simulink model "CDPR_simulation_w_motor"  (R2023b)
settings: Solver=ode15s  StartTime=0.0  StopTime=10.0  RelTol=1e-3
values from neighbouring files (symbols this model uses):
  A = 1e-6    (= 1e-06)    [init.m]
  a = [a1 a2 a3 a4]    [init.m]
  A_c_aug = [A_c    zeros(6,6) ... (first row only)    [init.m]
  b = [b1 b2 b3 b4]    [init.m]
  B_c_aug = [B_c; zeros(6,3)]    [init.m]
  d_c = [ 0 ... (first row only)    [init.m]
  d_c_aug = [d_c; zeros(6,1)]    [init.m]
  E = 100E9    (= 100000000000)    [init.m]
  f_max = 100    [init.m]
  f_min = 10    [init.m]
  f_ref = 25    [init.m]
  I_gain_f = 10    [init.m]
  Izz = 6.25e-4    (= 0.000625)    [init.m]
  K_a = [diag([-10,-10,-1]) zeros(3,3)]    [init.m]
  K_d = B_c\eye(6)    [init.m]
  K_f = [180*diag([1,1,1]) 10*diag([1,1,1])]    [init.m]
  K_r = pinv((B_c*K_f-A_c)\B_c)    [init.m]
  ln0 = zeros(size(b,2),1)    [init.m]
  mp = 0.250    (= 0.25)    [init.m]
  P_gain_f = 75    [init.m]
  q0 = [r0; theta0]    [init.m]
  qd0 = [xd0;yd0; thetad0]    [init.m]
  w = [ 0 ... (first row only)    [init.m]
  zeroI = [zeros(6,6);eye(6)]    [init.m]
undefined symbols (not defined in the file or in its folder): Clarke, current_m_max, current_m_min, fourier_coeff_a, fourier_coeff_b, i_m_max, i_m_min, J_m, K_e, l_m, n_p_pairs, r_m, r_w, thetar0
libraries: slpidlib x1
settings Model: Creator=Sølve  LastModifiedBy=solvno
settings DebuggingCC: UnconnectedInputMsg=warning  UnconnectedOutputMsg=warning  UnconnectedLineMsg=warning
settings ModelReferenceCC: EnableRefExpFcnMdlSchedulingChecks=on
settings RTWCC: DLArmComputeVersion=19.05

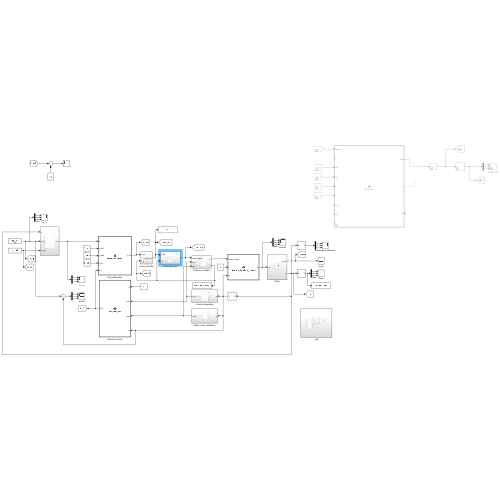
[thumbnail: Simulink's stored preview of the top-level diagram]
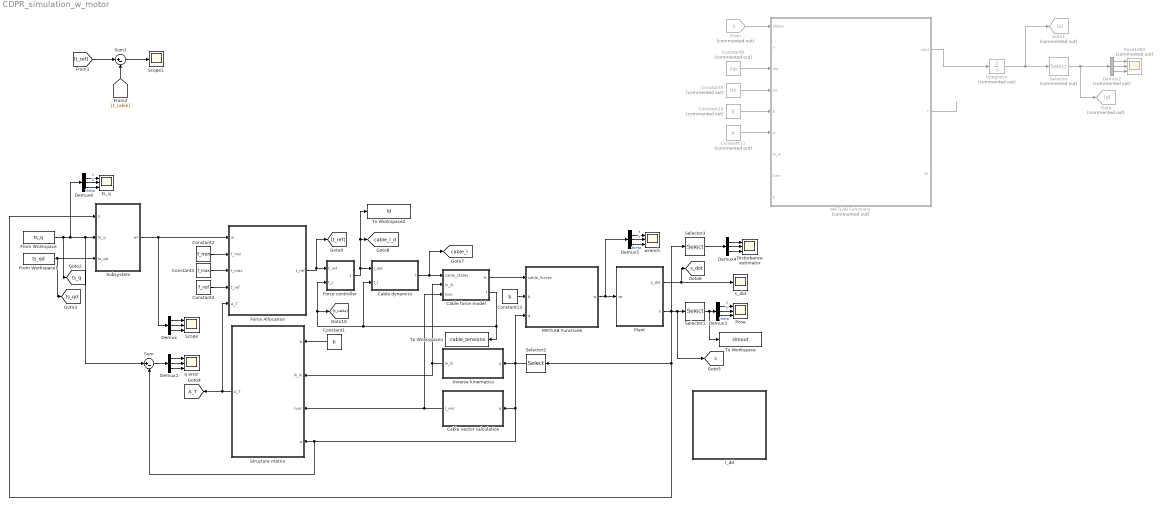
== system CDPR_simulation_w_motor ==
  Cable dynamics : Subsystem
  Cable force model : Subsystem
  Cable vector calculation : Subsystem
  Constant1 : Constant  Value=b
  Constant10 : Constant  Commented=on  Value=E
  Constant11 : Constant  Commented=on  Value=A
  Constant13 : Constant  Value=b
  Constant2 : Constant  Value=f_min
  Constant3 : Constant  Value=f_max
  Constant4 : Constant  Value=f_ref
  Constant8 : Constant  Commented=on  Value=mp
  Constant9 : Constant  Commented=on  Value=Izz
  Demux{,1,3..6} (6 alike) : Demux  Outputs=3
  Demux2 : Demux  Commented=on  Outputs=3
  Disturbance estimator : Scope  NumInputPorts=3
  Force Allocation : MATLAB Function  TreatAsAtomicUnit=on
  Force controller : Subsystem
  From : From  Commented=on  GotoTag=s
  From Workspace : FromWorkspace  VariableName=ts_q
  From Workspace1 : FromWorkspace  VariableName=ts_qd
  Goto : Goto  Commented=on  GotoTag=q
  Goto1 : Goto  Commented=on  GotoTag=s
  Integrator : Integrator  Commented=on  InitialCondition=[q0;qd0;ln0]
  Inverse kinematics : Subsystem
  MATLAB Function3 : MATLAB Function  Commented=on  TreatAsAtomicUnit=on
  MATLAB Function6 : MATLAB Function  TreatAsAtomicUnit=on
  Plant : Subsystem
  Pose : Scope  NumInputPorts=3
  Pose1000 : Scope  Commented=on  NumInputPorts=3
  Scope : Scope  NumInputPorts=3
  Scope1 : Scope
  Selector : Selector  Commented=on  InputPortWidth=10  IndexOptions=Index vector (dialog)  Indices=[1 2 3]  OutputSizes=1
  Selector1 : Selector  InputPortWidth=12  IndexOptions=Index vector (dialog)  Indices=[1 2 3]  OutputSizes=1
  Selector2 : Selector  InputPortWidth=12  IndexOptions=Index vector (dialog)  Indices=[1 2 3]  OutputSizes=1
  Selector3 : Selector  InputPortWidth=12  IndexOptions=Index vector (dialog)  Indices=[7 8 9]  OutputSizes=1
  Structure matrix : MATLAB Function  TreatAsAtomicUnit=on
  Subsystem : Subsystem
  Sum : Sum  Inputs=|+-
  Sum1 : Sum  Inputs=|+-
  To Workspace : ToWorkspace  VariableName=simout  SaveFormat=Timeseries  SampleTime=-1
  To Workspace1 : ToWorkspace  VariableName=cable_tensions  SaveFormat=Timeseries  SampleTime=-1
  To Workspace2 : ToWorkspace  VariableName=ld  SaveFormat=Timeseries  SampleTime=-1
  l_dd : Subsystem
  q error : Scope  NumInputPorts=3
  s_dot : Scope
  ts_q : Scope  NumInputPorts=3
  wrench : Scope  NumInputPorts=3
  tag scope: A_T=global, cable_l=global, cable_l_d=global, s=global, s_dot=global, ts_q=global, ts_qd=global
  wires:
  Constant1/1 -> Structure matrix/1(b)
  Constant2/1 -> Force Allocation/2(f_min)
  Constant4/1 -> Force Allocation/4(f_ref)
  Constant3/1 -> Force Allocation/3(f_max)
  Force Allocation/1(t_ref) -> Force controller/1(t_ref), [t_ref]
  Constant8/1 -> MATLAB Function3/3(mp)
  Constant9/1 -> MATLAB Function3/4(Izz)
  Constant10/1 -> MATLAB Function3/5(E)
  Constant11/1 -> MATLAB Function3/6(A)
  MATLAB Function3/2(t) -> ?
  MATLAB Function3/1(xdot) -> Integrator/1
  Integrator/1 -> Goto1/1, Selector/1
  Selector/1 -> Demux2/1, Goto/1
  From/1 -> MATLAB Function3/1(states)
  Inverse kinematics/1(ln_ik) -> Structure matrix/2(ln_ik), Cable force model/2(ln_ik)
  Demux/1 -> Scope/1
  Demux/2 -> Scope/2
  Demux/3 -> Scope/3
  Demux1/1 -> q error/1
  Demux1/3 -> q error/3
  Demux1/2 -> q error/2
  Selector2/1 -> Sum/2, Structure matrix/4(q), Cable vector calculation/1(q), MATLAB Function6/3(q), Inverse kinematics/1(q)
  Sum/1 -> Demux1/1
  Demux2/1 -> Pose1000/1
  Demux2/2 -> Pose1000/2
  Demux2/3 -> Pose1000/3
  Plant/2(s) -> Selector3/1, [s], Selector1/1, Subsystem/1(s), Selector2/1
  Demux3/3 -> Pose/3  "theta"
  Demux3/2 -> Pose/2  "y"
  Demux3/1 -> Pose/1  "x"
  Plant/1(s_dot) -> [s_dot], s_dot/1
  Constant13/1 -> MATLAB Function6/2(b)
  Cable force model/1(fc) -> MATLAB Function6/1(cable_forces)
  Cable dynamics/1(l) -> [cable_l], Cable force model/1(cable_states)
  Cable force model/2(t) -> Cable dynamics/2(t_l), Force controller/2(t_c), [t_cable], To Workspace1/1
  Cable vector calculation/1(l_vec) -> Cable force model/3(lvec), Structure matrix/3(lvec)
  Structure matrix/1(A_T) -> [A_T], Force Allocation/5(A_T)
  Selector1/1 -> To Workspace/1, Demux3/1
  Subsystem/1(wr) -> Demux/1, Force Allocation/1(w)
  From Workspace1/1 -> [ts_qd], Subsystem/3(ts_qd)
  Selector3/1 -> Demux4/1
  Demux4/1 -> Disturbance estimator/1
  Demux4/2 -> Disturbance estimator/2
  Demux4/3 -> Disturbance estimator/3
  Demux5/1 -> wrench/1  "x"
  Demux5/3 -> wrench/3  "theta"
  Demux5/2 -> wrench/2  "y"
  MATLAB Function6/1(w) -> Demux5/1, Plant/1(wr)
  [t_cable] -> Sum1/2
  [t_ref] -> Sum1/1
  Sum1/1 -> Scope1/1
  Force controller/1(l_dot_ref) -> To Workspace2/1, [cable_l_d], Cable dynamics/1(l_dot)
  Demux6/1 -> ts_q/1  "x"
  Demux6/3 -> ts_q/3  "theta"
  Demux6/2 -> ts_q/2  "y"
  From Workspace/1 -> Demux6/1, Subsystem/2(ts_q), Sum/1, [ts_q]

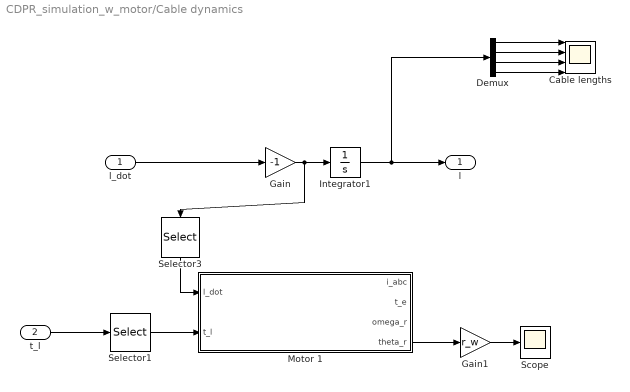
== system CDPR_simulation_w_motor/Cable dynamics ==
  l_dot : Inport
  t_l : Inport  Port=2
  Cable lengths : Scope  NumInputPorts=4
  Demux : Demux
  Gain : Gain  Gain=-1
  Gain1 : Gain  Gain=r_w
  Integrator1 : Integrator  InitialCondition=ln0
  Motor 1 : Subsystem
  Scope : Scope
  Selector1 : Selector  InputPortWidth=4  IndexOptions=Index vector (dialog)  Indices=[1]  OutputSizes=1
  Selector3 : Selector  InputPortWidth=4  IndexOptions=Index vector (dialog)  Indices=[1]  OutputSizes=1
  l : Outport
  wires:
  Integrator1/1 -> Demux/1, l/1
  l_dot/1 -> Gain/1
  Gain/1 -> Selector3/1, Integrator1/1
  Demux/1 -> Cable lengths/1
  Demux/2 -> Cable lengths/2
  Demux/3 -> Cable lengths/3
  Demux/4 -> Cable lengths/4
  t_l/1 -> Selector1/1
  Motor 1/4(theta_r) -> Gain1/1
  Gain1/1 -> Scope/1
  Selector3/1 -> Motor 1/1(l_dot)
  Selector1/1 -> Motor 1/2(t_l)

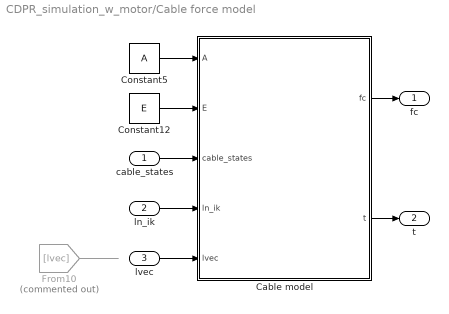
== system CDPR_simulation_w_motor/Cable force model ==
  cable_states : Inport
  ln_ik : Inport  Port=2
  lvec : Inport  Port=3
  Cable model : MATLAB Function  TreatAsAtomicUnit=on
  Constant12 : Constant  Value=E
  Constant5 : Constant  Value=A
  From10 : From  Commented=on  GotoTag=lvec  TagVisibility=global
  fc : Outport
  t : Outport  Port=2
  wires:
  Constant12/1 -> Cable model/2(E)
  From10/1 -> ?
  ln_ik/1 -> Cable model/4(ln_ik)
  Constant5/1 -> Cable model/1(A)
  Cable model/2(t) -> t/1
  cable_states/1 -> Cable model/3(cable_states)
  Cable model/1(fc) -> fc/1
  lvec/1 -> Cable model/5(lvec)

== system CDPR_simulation_w_motor/Cable vector calculation ==
  q : Inport
  Constant : Constant  Value=b
  Constant5 : Constant  Value=a
  MATLAB Function5 : MATLAB Function  TreatAsAtomicUnit=on
  l_vec : Outport
  wires:
  Constant/1 -> MATLAB Function5/3(b)
  q/1 -> MATLAB Function5/1(q)
  Constant5/1 -> MATLAB Function5/2(a)
  MATLAB Function5/1(l_vec) -> l_vec/1

== system CDPR_simulation_w_motor/Force controller ==
  t_ref : Inport
  t_c : Inport  Port=2
  PID Controller (2DOF) : slpidlib/PID Controller (2DOF)  Controller=PI  Form=Parallel  TimeDomain=Continuous-time  UseExternalTs=off  SampleTime=-1  IntegratorMethod=Forward Euler  FilterMethod=Forward Euler  ControllerParametersSource=internal  P=P_gain_f  I=I_gain_f  UseKiTs=off  D=5  N=100  UseFilter=on  b=1  c=1  TunerSelectOption=Transfer Function Based (PID Tuner App)  InitialConditionSource=internal  InitialConditionForIntegrator=0  InitialConditionForFilter=0  DifferentiatorICPrevScaledInput=0  ExternalReset=none  TrackingMode=off  Kt=1  LimitOutput=off  SatLimitsSource=internal  UpperSaturationLimit=inf  LowerSaturationLimit=-inf  LinearizeAsGain=on  AntiWindupMode=none  Kb=1  LimitIntegrator=off  UpperIntegratorSaturationLimit=inf  LowerIntegratorSaturationLimit=-inf  POutMin=[]  POutMax=[]  IOutMin=[]  IOutMax=[]  DOutMin=[]  DOutMax=[]  NOutMin=[]  NOutMax=[]  bOutMin=[]  bOutMax=[]  cOutMin=[]  cOutMax=[]  SumOutMin=[]  SumOutMax=[]  SaturationOutMin=[]  SaturationOutMax=[]  PParamMin=[]  PParamMax=[]  IParamMin=[]  IParamMax=[]  DParamMin=[]  DParamMax=[]  NParamMin=[]  NParamMax=[]  bParamMin=[]  bParamMax=[]  cParamMin=[]  cParamMax=[]  KbParamMin=[]  KbParamMax=[]  KtParamMin=[]  KtParamMax=[]  KbOutMin=[]  KbOutMax=[]  KtOutMin=[]  KtOutMax=[]  IntegratorOutMin=[]  IntegratorOutMax=[]  FilterOutMin=[]  FilterOutMax=[]  SumI1OutMin=[]  SumI1OutMax=[]  SumI2OutMin=[]  SumI2OutMax=[]  SumI3OutMin=[]  SumI3OutMax=[]  SumI4OutMin=[]  SumI4OutMax=[]  SumDOutMin=[]  SumDOutMax=[]  Sum1OutMin=[]  Sum1OutMax=[]  Sum2OutMin=[]  Sum2OutMax=[]  Sum3OutMin=[]  Sum3OutMax=[]  DifferentiatorOutMin=[]  DifferentiatorOutMax=[]  FilterDiffOutCoefMin=[]  FilterDiffOutCoefMax=[]  ReciprocalOutMin=[]  ReciprocalOutMax=[]  SumDenOutMin=[]  SumDenOutMax=[]  SumNumOutMin=[]  SumNumOutMax=[]  DivideOutMin=[]  DivideOutMax=[]  UdiffTsProdOutMin=[]  UdiffTsProdOutMax=[]  NTsProdOutMin=[]  NTsProdOutMax=[]  UintegralTsProdOutMin=[]  UintegralTsProdOutMax=[]  UngainTsProdOutMin=[]  UngainTsProdOutMax=[]  ClampingZeroOutDataTypeStr=Inherit: Inherit via back propagation  ClampingZeroOutMin=[]  ClampingZeroOutMax=[]  FilterDenConstantOutDataTypeStr=Inherit: Inherit via back propagation  FilterDenConstantOutMin=[]  FilterDenConstantOutMax=[]  PCopyOutDataTypeStr=Inherit: Inherit via back propagation  PCopyOutMin=[]  PCopyOutMax=[]  NCopyOutDataTypeStr=Inherit: Inherit via back propagation  NCopyOutMin=[]  NCopyOutMax=[]  IntegratorContinuousStateAttributes=''  IntegratorStateMustResolveToSignalObject=off  IntegratorRTWStateStorageClass=Auto  FilterContinuousStateAttributes=''  FilterStateMustResolveToSignalObject=off  FilterRTWStateStorageClass=Auto  ParallelPVariant=InternalParameters  IdealPVariant=Disabled  IVariant=InternalParameters  DVariant=Disabled  bVariant=InternalParameters  cVariant=Disabled  IntegratorVariant=Continuous  SatVariant=Disabled  AWVariant=Passthrough  PCopyVariant=Disabled  TRVariant=Disabled  FdbkBlocksVariant=Forward  IdealPFdbkVariant=Disabled  SatFdbkVariant=Disabled  DerivativeFilterVariant=Disabled  NVariant=Disabled  NCopyVariant=Disabled_SignalSpec  FilterICVariant=Disabled  IntegratorICVariant=InternalICs  ExternalResetVariant=Disabled  TRSumVariant=Passthrough  SumFdbkVariant=Disabled  SumVariant=Sum_PI  TsampFilterVariant=InternalTs  TsampNgainVariant=Passthrough  TsampIntegralVariant=Disabled_SignalSpec  ExternalSaturationOutDataTypeStr=Inherit: Same as second input
  Saturation : Saturate  UpperLimit=5  LowerLimit=-5
  l_dot_ref : Outport
  wires:
  t_ref/1 -> PID Controller (2DOF)/1
  t_c/1 -> PID Controller (2DOF)/2
  PID Controller (2DOF)/1 -> Saturation/1
  Saturation/1 -> l_dot_ref/1

== system CDPR_simulation_w_motor/Inverse kinematics ==
  q : Inport
  Constant6 : Constant  Value=a
  Constant7 : Constant  Value=b
  MATLAB Function4 : MATLAB Function  TreatAsAtomicUnit=on
  ln_ik : Outport
  wires:
  MATLAB Function4/1(ln) -> ln_ik/1
  Constant6/1 -> MATLAB Function4/2(a)
  q/1 -> MATLAB Function4/1(q)
  Constant7/1 -> MATLAB Function4/3(b)

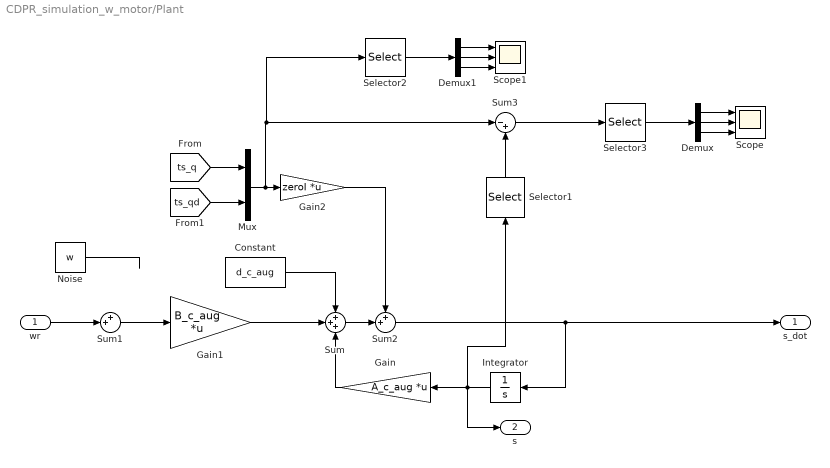
== system CDPR_simulation_w_motor/Plant ==
  wr : Inport
  Constant : Constant  Value=d_c_aug
  Demux : Demux  Outputs=3
  Demux1 : Demux  Outputs=3
  Gain : Gain  Gain=A_c_aug  Multiplication=Matrix(K*u)
  Gain1 : Gain  Gain=B_c_aug  Multiplication=Matrix(K*u)
  Gain2 : Gain  Gain=zeroI  Multiplication=Matrix(K*u)
  Integrator : Integrator  InitialCondition=[q0;qd0; zeros(6,1)]
  Mux : Mux  Inputs=2
  Noise : Constant  Value=w
  Scope : Scope  NumInputPorts=3
  Scope1 : Scope  NumInputPorts=3
  Selector1 : Selector  InputPortWidth=12  IndexOptions=Index vector (dialog)  Indices=[1 2 3 4 5 6]  OutputSizes=1
  Selector2 : Selector  InputPortWidth=6  IndexOptions=Index vector (dialog)  Indices=[1 2 3]  OutputSizes=1
  Selector3 : Selector  InputPortWidth=6  IndexOptions=Index vector (dialog)  Indices=[1 2 3]  OutputSizes=1
  Sum : Sum  Inputs=+++
  Sum1 : Sum  Inputs=++|
  Sum2 : Sum  Inputs=++|
  Sum3 : Sum  Inputs=|-+
  s_dot : Outport
  s : Outport  Port=2
  wires:
  Integrator/1 -> Selector1/1, s/1, Gain/1
  wr/1 -> Sum1/2
  Constant/1 -> Sum/1
  Gain1/1 -> Sum/2
  Gain/1 -> Sum/3
  Sum2/1 -> Integrator/1, s_dot/1
  [ts_q] -> Mux/1
  [ts_qd] -> Mux/2
  Sum1/1 -> Gain1/1
  Noise/1 -> ?
  Sum/1 -> Sum2/2
  Gain2/1 -> Sum2/1
  Sum3/1 -> Selector3/1
  Demux/1 -> Scope/1
  Demux/2 -> Scope/2
  Demux/3 -> Scope/3
  Selector3/1 -> Demux/1
  Selector1/1 -> Sum3/2
  Demux1/3 -> Scope1/3
  Selector2/1 -> Demux1/1
  Demux1/2 -> Scope1/2
  Demux1/1 -> Scope1/1
  Mux/1 -> Selector2/1, Sum3/1, Gain2/1

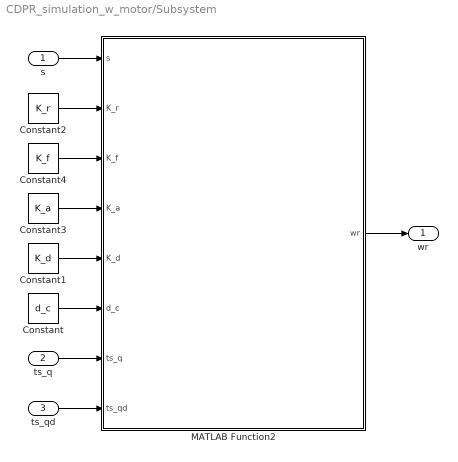
== system CDPR_simulation_w_motor/Subsystem ==
  s : Inport
  ts_q : Inport  Port=2
  ts_qd : Inport  Port=3
  Constant : Constant  Value=d_c
  Constant1 : Constant  Value=K_d
  Constant2 : Constant  Value=K_r
  Constant3 : Constant  Value=K_a
  Constant4 : Constant  Value=K_f
  MATLAB Function2 : MATLAB Function  TreatAsAtomicUnit=on
  wr : Outport
  wires:
  ts_q/1 -> MATLAB Function2/7(ts_q)
  ts_qd/1 -> MATLAB Function2/8(ts_qd)
  MATLAB Function2/1(wr) -> wr/1
  s/1 -> MATLAB Function2/1(s)
  Constant/1 -> MATLAB Function2/6(d_c)
  Constant1/1 -> MATLAB Function2/5(K_d)
  Constant2/1 -> MATLAB Function2/2(K_r)
  Constant3/1 -> MATLAB Function2/4(K_a)
  Constant4/1 -> MATLAB Function2/3(K_f)

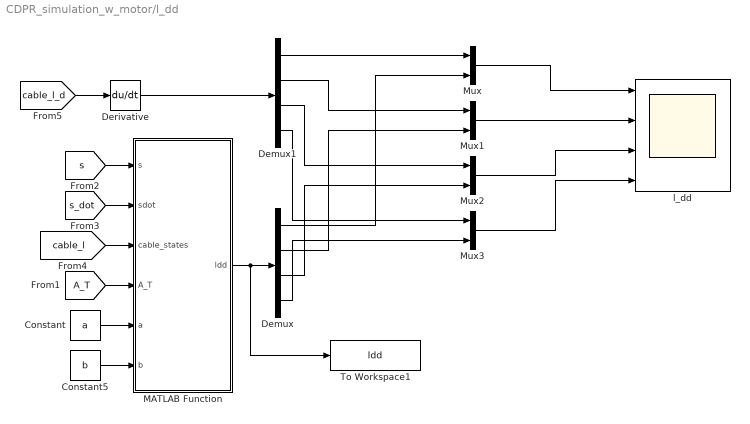
== system CDPR_simulation_w_motor/l_dd ==
  Constant : Constant  Value=a
  Constant5 : Constant  Value=b
  Demux : Demux
  Demux1 : Demux
  Derivative : Derivative  CoefficientInTFapproximation=0.0001
  MATLAB Function : MATLAB Function  TreatAsAtomicUnit=on
  Mux{,1..3} (4 alike) : Mux  Inputs=2
  To Workspace1 : ToWorkspace  VariableName=ldd  SaveFormat=Timeseries  SampleTime=-1
  l_dd : Scope  NumInputPorts=4
  wires:
  Constant/1 -> MATLAB Function/5(a)
  [A_T] -> MATLAB Function/4(A_T)
  [cable_l_d] -> Derivative/1
  Constant5/1 -> MATLAB Function/6(b)
  [s] -> MATLAB Function/1(s)
  [cable_l] -> MATLAB Function/3(cable_states)
  [s_dot] -> MATLAB Function/2(sdot)
  MATLAB Function/1(ldd) -> To Workspace1/1, Demux/1
  Derivative/1 -> Demux1/1
  Demux1/1 -> Mux/1
  Demux/1 -> Mux/2
  Demux1/2 -> Mux1/1
  Demux/2 -> Mux1/2
  Demux/3 -> Mux2/2
  Demux1/3 -> Mux2/1
  Demux1/4 -> Mux3/1
  Demux/4 -> Mux3/2
  Mux/1 -> l_dd/1
  Mux1/1 -> l_dd/2
  Mux2/1 -> l_dd/3
  Mux3/1 -> l_dd/4

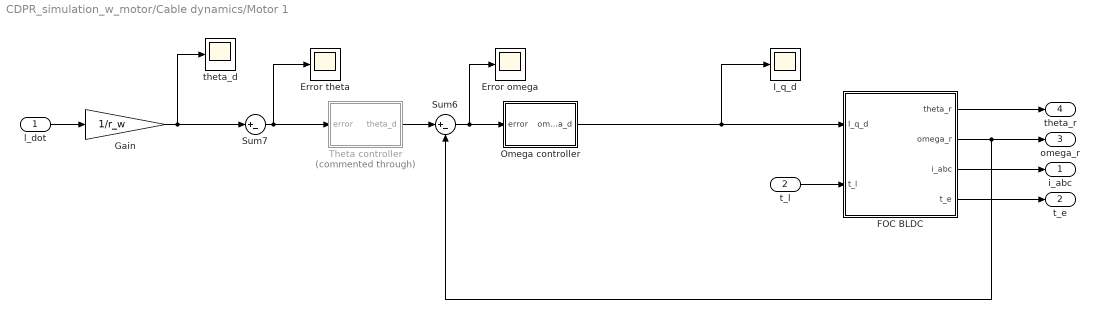
== system CDPR_simulation_w_motor/Cable dynamics/Motor 1 ==
  l_dot : Inport
  t_l : Inport  Port=2
  Error omega : Scope
  Error theta : Scope
  FOC BLDC : Subsystem
  Gain : Gain  Gain=1/r_w
  I_q_d : Scope
  Omega controller : Subsystem
  Sum6 : Sum  Inputs=|+-
  Sum7 : Sum  Inputs=|+-
  Theta controller : Subsystem  Commented=through
  theta_d : Scope
  i_abc : Outport
  t_e : Outport  Port=2
  omega_r : Outport  Port=3
  theta_r : Outport  Port=4
  wires:
  FOC BLDC/2(omega_r) -> Sum6/2, omega_r/1
  FOC BLDC/3(i_abc) -> i_abc/1
  Sum7/1 -> Theta controller/1(error), Error theta/1
  Sum6/1 -> Omega controller/1(error), Error omega/1
  FOC BLDC/1(theta_r) -> theta_r/1
  Theta controller/1(theta_d) -> Sum6/1
  FOC BLDC/4(t_e) -> t_e/1
  Omega controller/1(omega_d) -> I_q_d/1, FOC BLDC/1(I_q_d)
  l_dot/1 -> Gain/1
  t_l/1 -> FOC BLDC/2(t_l)
  Gain/1 -> theta_d/1, Sum7/1

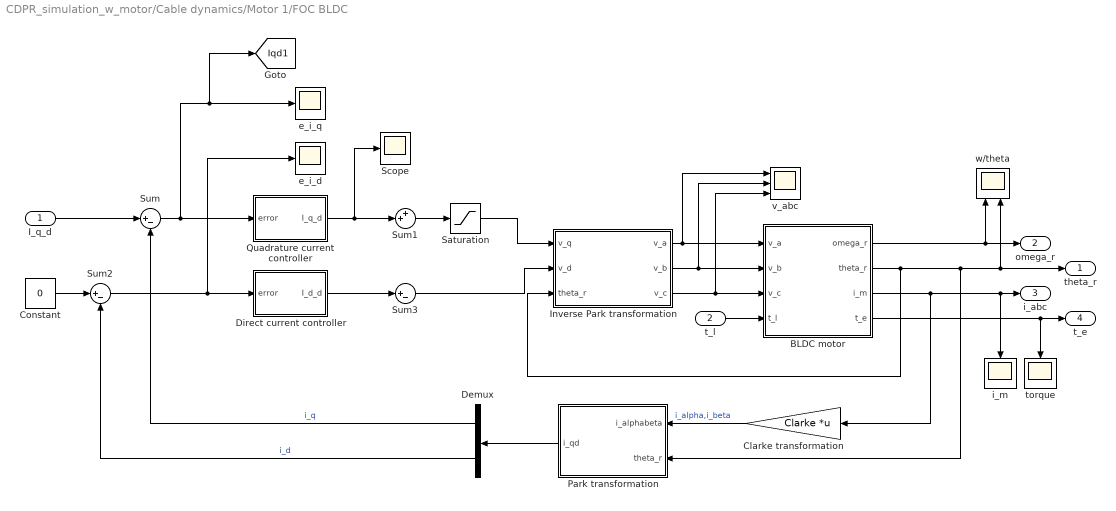
== system CDPR_simulation_w_motor/Cable dynamics/Motor 1/FOC BLDC ==
  I_q_d : Inport
  t_l : Inport  Port=2
  BLDC motor : Subsystem
  Clarke transformation : Gain  Gain=Clarke  Multiplication=Matrix(K*u) (u vector)
  Constant : Constant  Value=0
  Demux : Demux  Outputs=2
  Direct current controller : Subsystem
  Inverse Park transformation : MATLAB Function  TreatAsAtomicUnit=on
  Park transformation : MATLAB Function  TreatAsAtomicUnit=on
  Quadrature current controller : Subsystem
  Saturation : Saturate  UpperLimit=i_m_max  LowerLimit=i_m_min
  Scope : Scope
  Sum : Sum  Inputs=|+-
  Sum1 : Sum  Inputs=++|
  Sum2 : Sum  Inputs=|+-
  Sum3 : Sum  Inputs=|+-
  e_i_d : Scope
  e_i_q : Scope
  i_m : Scope
  torque : Scope
  v_abc : Scope  NumInputPorts=3
  w/theta : Scope  NumInputPorts=2
  theta_r : Outport
  omega_r : Outport  Port=2
  i_abc : Outport  Port=3
  t_e : Outport  Port=4
  tag scope: Iqd1=global
  wires:
  Sum/1 -> Quadrature current controller/1(error), [Iqd1], e_i_q/1
  Quadrature current controller/1(I_q_d) -> Scope/1, Sum1/2
  Constant/1 -> Sum2/1
  Sum2/1 -> Direct current controller/1(error), e_i_d/1
  Direct current controller/1(I_d_d) -> Sum3/1
  Sum1/1 -> Saturation/1
  Sum3/1 -> Inverse Park transformation/2(v_d)
  Inverse Park transformation/1(v_a) -> v_abc/1, BLDC motor/1(v_a)
  Inverse Park transformation/2(v_b) -> v_abc/2, BLDC motor/2(v_b)
  Inverse Park transformation/3(v_c) -> v_abc/3, BLDC motor/3(v_c)
  t_l/1 -> BLDC motor/4(t_l)
  BLDC motor/1(omega_r) -> omega_r/1, w/theta/1
  Clarke transformation/1 -> Park transformation/1(i_alphabeta)  "i_alpha,i_beta"
  BLDC motor/2(theta_r) -> Park transformation/2(theta_r), theta_r/1, w/theta/2, Inverse Park transformation/3(theta_r)
  Park transformation/1(i_qd) -> Demux/1
  Demux/1 -> Sum/2  "i_q"
  Demux/2 -> Sum2/2  "i_d"
  BLDC motor/3(i_m) -> i_m/1, i_abc/1, Clarke transformation/1
  BLDC motor/4(t_e) -> torque/1, t_e/1
  I_q_d/1 -> Sum/1
  Saturation/1 -> Inverse Park transformation/1(v_q)

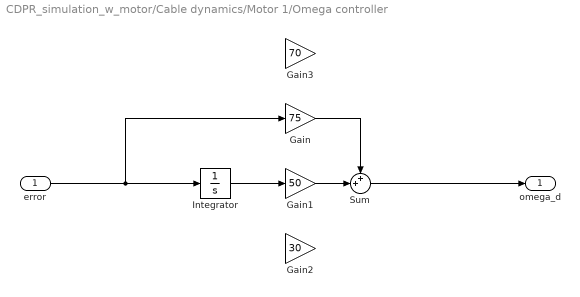
== system CDPR_simulation_w_motor/Cable dynamics/Motor 1/Omega controller ==
  error : Inport
  Gain : Gain  Gain=75
  Gain1 : Gain  Gain=50
  Gain2 : Gain  Gain=30
  Gain3 : Gain  Gain=70
  Integrator : Integrator
  Sum : Sum  Inputs=++|
  omega_d : Outport
  wires:
  Sum/1 -> omega_d/1
  Gain/1 -> Sum/1
  Gain1/1 -> Sum/2
  Integrator/1 -> Gain1/1
  error/1 -> Integrator/1, Gain/1

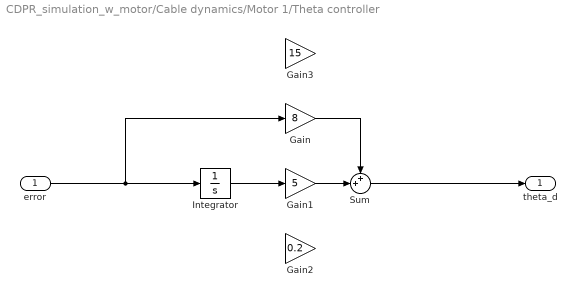
== system CDPR_simulation_w_motor/Cable dynamics/Motor 1/Theta controller ==
  error : Inport
  Gain : Gain  Gain=8
  Gain1 : Gain  Gain=5
  Gain2 : Gain  Gain=0.2
  Gain3 : Gain  Gain=15
  Integrator : Integrator
  Sum : Sum  Inputs=++|
  theta_d : Outport
  wires:
  error/1 -> Gain/1, Integrator/1
  Integrator/1 -> Gain1/1
  Gain1/1 -> Sum/2
  Gain/1 -> Sum/1
  Sum/1 -> theta_d/1

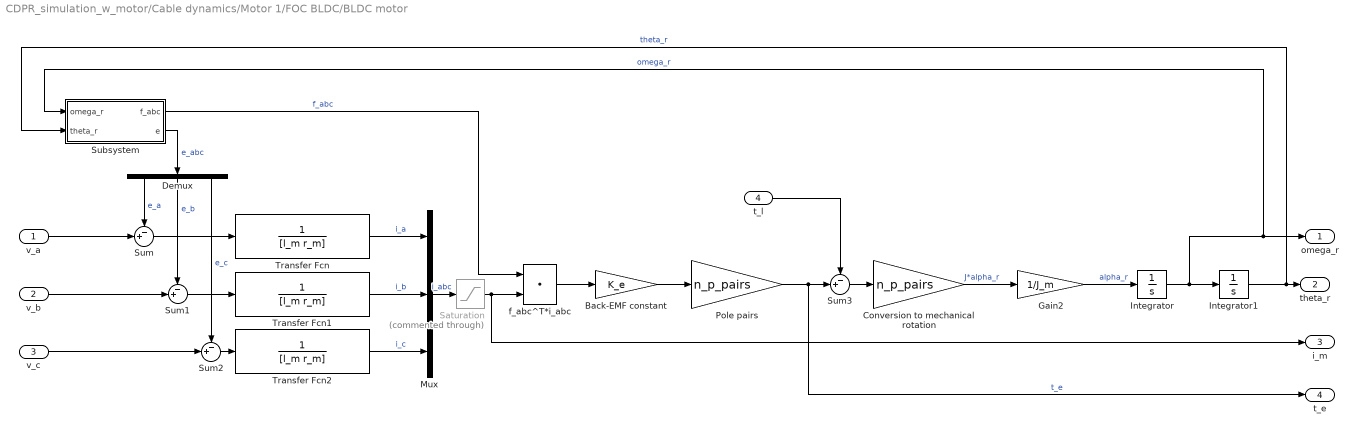
== system CDPR_simulation_w_motor/Cable dynamics/Motor 1/FOC BLDC/BLDC motor ==
  v_a : Inport
  v_b : Inport  Port=2
  v_c : Inport  Port=3
  t_l : Inport  Port=4
  Back-EMF constant : Gain  Gain=K_e
  Conversion to mechanical rotation : Gain  Gain=n_p_pairs
  Demux : Demux  Outputs=3
  Gain2 : Gain  Gain=1/J_m
  Integrator : Integrator  InitialCondition=0.001
  Integrator1 : Integrator  InitialCondition=thetar0(1)
  Mux : Mux  Inputs=3
  Pole pairs : Gain  Gain=n_p_pairs
  Saturation : Saturate  Commented=through  UpperLimit=current_m_max  LowerLimit=current_m_min
  Subsystem : Subsystem
  Sum{,1..3} (4 alike) : Sum  Inputs=-+|
  Transfer Fcn : TransferFcn  Denominator=[l_m r_m]
  Transfer Fcn1 : TransferFcn  Denominator=[l_m r_m]
  Transfer Fcn2 : TransferFcn  Denominator=[l_m r_m]
  f_abc^T*i_abc : DotProduct  OutDataTypeStr=Inherit: Inherit via internal rule
  omega_r : Outport
  theta_r : Outport  Port=2
  i_m : Outport  Port=3
  t_e : Outport  Port=4
  wires:
  v_a/1 -> Sum/2
  v_b/1 -> Sum1/2
  v_c/1 -> Sum2/2
  Demux/1 -> Sum/1  "e_a"
  Demux/2 -> Sum1/1  "e_b"
  Demux/3 -> Sum2/1  "e_c"
  Subsystem/2(e) -> Demux/1  "e_abc"
  Sum/1 -> Transfer Fcn/1
  Sum1/1 -> Transfer Fcn1/1
  Sum2/1 -> Transfer Fcn2/1
  Transfer Fcn2/1 -> Mux/3  "i_c"
  Transfer Fcn1/1 -> Mux/2  "i_b"
  Transfer Fcn/1 -> Mux/1  "i_a"
  Subsystem/1(f_abc) -> f_abc^T*i_abc/1  "f_abc"
  Sum3/1 -> Conversion to mechanical rotation/1
  f_abc^T*i_abc/1 -> Back-EMF constant/1
  Back-EMF constant/1 -> Pole pairs/1
  t_l/1 -> Sum3/1
  Gain2/1 -> Integrator/1  "alpha_r"
  Integrator/1 -> Subsystem/1(omega_r), omega_r/1, Integrator1/1  "omega_r"
  Integrator1/1 -> Subsystem/2(theta_r), theta_r/1  "theta_r"
  Pole pairs/1 -> t_e/1, Sum3/2  "t_e"
  Mux/1 -> Saturation/1  "i_abc"
  Saturation/1 -> f_abc^T*i_abc/2, i_m/1
  Conversion to mechanical rotation/1 -> Gain2/1  "J*alpha_r"

== system CDPR_simulation_w_motor/Cable dynamics/Motor 1/FOC BLDC/Direct current controller ==
  error : Inport
  Gain : Gain  Gain=100
  Gain1 : Gain  Gain=70
  Integrator : Integrator
  Sum : Sum  Inputs=++|
  I_d_d : Outport
  wires:
  error/1 -> Gain/1, Integrator/1
  Integrator/1 -> Gain1/1
  Gain1/1 -> Sum/2
  Gain/1 -> Sum/1
  Sum/1 -> I_d_d/1

== system CDPR_simulation_w_motor/Cable dynamics/Motor 1/FOC BLDC/Quadrature current controller ==
  error : Inport
  Gain : Gain  Gain=40
  Gain1 : Gain  Gain=50
  Integrator : Integrator
  Sum : Sum  Inputs=++|
  I_q_d : Outport
  wires:
  Sum/1 -> I_q_d/1
  Gain/1 -> Sum/1
  Gain1/1 -> Sum/2
  Integrator/1 -> Gain1/1
  error/1 -> Integrator/1, Gain/1

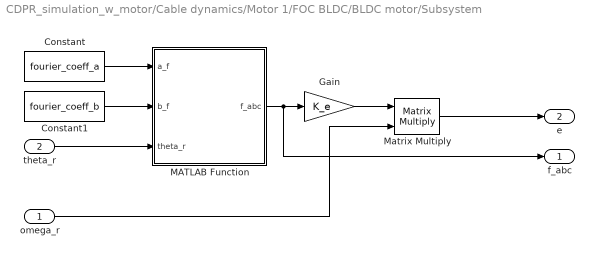
== system CDPR_simulation_w_motor/Cable dynamics/Motor 1/FOC BLDC/BLDC motor/Subsystem ==
  omega_r : Inport
  theta_r : Inport  Port=2
  Constant : Constant  Value=fourier_coeff_a
  Constant1 : Constant  Value=fourier_coeff_b
  Gain : Gain  Gain=K_e
  MATLAB Function : MATLAB Function  TreatAsAtomicUnit=on
  Matrix Multiply : Product  Multiplication=Matrix(*)
  f_abc : Outport
  e : Outport  Port=2
  wires:
  theta_r/1 -> MATLAB Function/3(theta_r)
  Constant/1 -> MATLAB Function/1(a_f)
  Constant1/1 -> MATLAB Function/2(b_f)
  MATLAB Function/1(f_abc) -> f_abc/1, Gain/1
  Gain/1 -> Matrix Multiply/1
  omega_r/1 -> Matrix Multiply/2
  Matrix Multiply/1 -> e/1

== matlab function CDPR_simulation_w_motor/MATLAB Function6 ==
  data: cable_forces input; w output; b input; q input
function w = calculate_resultant_forces(cable_forces, b, q)
theta = q(3);
R = R_z(theta);
m = zeros(1,4);
for i = 1:4
    cross_prod = cross([R*b(:,i);0],[cable_forces(:,i);0]);
    m(i) = cross_prod(3);
end

f_res = sum(cable_forces,2);
m_res = sum(m, 2);
% M_res = m(1) + m(2) + m(3) + m(4);
w = [f_res;m_res];
% y = u;

== matlab function CDPR_simulation_w_motor/l_dd/MATLAB Function ==
  data: s input; ldd output; sdot input; cable_states input; A_T input; a input; b input
function ldd = fcn(s, sdot, cable_states, A_T, a, b)
% Positions
x     = s(1);
y     = s(2);
theta = s(3);

q = [x;y;theta];

% Velocities
xd     = s(4);
yd     = s(5);
thetad = s(6);

qd = [xd;yd;thetad];

% Accelerations
xdd     = sdot(4);
ydd     = sdot(5);
thetadd = sdot(6);

qdd = [xdd; ydd; thetadd];

r   = [x;y];
rd  = [xd;yd];
rdd = [xdd;ydd];

% Cable lengths
l = [cable_states(1); cable_states(2); cable_states(3); cable_states(4)];

% Norms of the derivative of cable lengths
ldn = -A_T.'*qd;

thetadskew = [0 -thetad; thetad 0];
thetaddskew = [0 -thetadd; thetadd 0];

u = calculate_uvec(q,a,b);

R = R_z(theta);

ldd = zeros(4,1);
ldd(1) = - u(:,1).' ... % u1^T
      * (rdd + R*thetadskew*thetadskew*b(:,1) + R*thetaddskew*b(:,1)) ... % r_dd + b_i_dd
      - 1/l(1)^2*((r + R*b(:,1)-a(:,1))*ldn(1) - (rd + R*thetadskew*b(:,1))*l(1)).' ... % u_d^T
      * (rd + R*b(:,1)); % r_d + b_i_d
ldd(2) = - u(:,2).' ... % u2^T
      * (rdd + R*thetadskew*thetadskew*b(:,2) + R*thetaddskew*b(:,2)) ... % r_dd + b_i_dd
      - 1/l(2)^2*((r + R*b(:,2)-a(:,2))*ldn(2) - (rd + R*thetadskew*b(:,2))*l(2)).' ... % u_d^T
      * (rd + R*b(:,2)); % r_d + b_i_d
ldd(3) = - u(:,3).' ... % u3^T
      * (rdd + R*thetadskew*thetadskew*b(:,3) + R*thetaddskew*b(:,3)) ... % r_dd + b_i_dd
      - 1/l(3)^2*((r + R*b(:,3)-a(:,3))*ldn(3) - (rd + R*thetadskew*b(:,3))*l(3)).' ... % u_d^T
      * (rd + R*b(:,3)); % r_d + b_i_d
ldd(4) = - u(:,4).' ... % u4^T
      * (rdd + R*thetadskew*thetadskew*b(:,4) + R*thetaddskew*b(:,4)) ... % r_dd + b_i_dd
      - 1/l(4)^2*((r + R*b(:,4)-a(:,4))*ldn(4) - (rd + R*thetadskew*b(:,4))*l(4)).' ... % u_d^T
      * (rd + R*b(:,4)); % r_d + b_i_d
ldd = -ldd;
% y = u;

== matlab function CDPR_simulation_w_motor/Cable dynamics/Motor 1/FOC BLDC/BLDC motor/Subsystem/MATLAB Function ==
  data: a_f input; f_abc output; b_f input; theta_r input
function f_abc  = normalized_back_EMF(a_f,b_f,theta_r)
sa = 0;
sb = 0;
sc = 0;
ca = 0;
cb = 0;
cc = 0;
n = size(a_f,1);

for i = 1:n
%     ca = ca + a(i,1)*cos((i-1)*theta_r);
    cb = cb + a_f(i,2)*cos((i-1)*theta_r);
    cc = cc + a_f(i,3)*cos((i-1)*theta_r); 
end
for i = 1:2:n
    sa = sa + b_f(i,1)*sin(i*theta_r);
    sb = sb + b_f(i,2)*sin(i*theta_r);
    sc = sc + b_f(i,3)*sin(i*theta_r);
end
f_a = ca+sa;
f_b = cb+sb;
f_c = cc+sc;

f_abc = [f_a;f_b;f_c];

== matlab function CDPR_simulation_w_motor/Cable dynamics/Motor 1/FOC BLDC/Inverse Park transformation ==
  data: v_q input; v_d input; v_a output; theta_r input; v_b output; v_c output
function [v_a, v_b, v_c] = inverse_park(v_q, v_d, theta_r)
Park_inv = [cos(theta_r)          -sin(theta_r);
            cos(theta_r - 2*pi/3) -sin(theta_r - 2*pi/3);
            cos(theta_r + 2*pi/3) -sin(theta_r + 2*pi/3)];

v_abc = Park_inv*[v_d;v_q];

v_a = v_abc(1);
v_b = v_abc(2);
v_c = v_abc(3);

== matlab function CDPR_simulation_w_motor/Cable dynamics/Motor 1/FOC BLDC/Park transformation ==
  data: i_alphabeta input; i_qd output; theta_r input
function i_qd  = park(i_alphabeta, theta_r)
Park = [-sin(theta_r) cos(theta_r);
         cos(theta_r) sin(theta_r)];
i_qd = Park*i_alphabeta;

== matlab function CDPR_simulation_w_motor/Force Allocation ==
  data: w input; f_min input; f_max input; f_ref input; A_T input; t_ref output
function t_ref = force_allocation(w, f_min, f_max, f_ref, A_T)
coder.extrinsic('quadprog');
coder.extrinsic('optimoptions');
options = optimoptions('quadprog','Display','off');
t_ref = zeros(4,1);
t_ref = quadprog(eye(4),-f_ref*ones(4,1), ...
                 [],[], ...
                 A_T, w, ...
                 f_min*ones(4,1),f_max*ones(4,1), ...
                 [], options);

== matlab function CDPR_simulation_w_motor/Structure matrix ==
  data: b input; ln_ik input; lvec input; q input; A_T output
function A_T = calculate_sm(b, ln_ik, lvec, q)
    theta = q(3);

%     ln = inverse_kinematics(a, b, q, 4);
%     l = calculate_l_vec(q, a, b);
    u = [lvec(:,1)/ln_ik(1) lvec(:,2)/ln_ik(2) lvec(:,3)/ln_ik(3) lvec(:,4)/ln_ik(4)];

    R = R_z(theta);
    bi = [R*b(:,1) R*b(:,2) R*b(:,3) R*b(:,4)];
    
    bcrossu = zeros(1,4);
    for i = 1:4
        biskew = skew([bi(:,i); 0]);
        crossProd = biskew*[u(:,i);0];
        bcrossu(i) = crossProd(3);
    end
    
    A_T = [u;bcrossu];
end

function uskew = skew(u)
    u1 = u(1);
    u2 = u(2);
    u3 = u(3);
    uskew = [ 0  -u3  u2;
              u3  0  -u1;
             -u2  u1  0];
end

== matlab function CDPR_simulation_w_motor/Subsystem/MATLAB Function2 ==
  data: s input; K_r input; K_f input; K_a input; K_d input; d_c input; wr output; ts_q input; ts_qd input
function wr = controller(s, K_r, K_f, K_a, K_d, d_c, ts_q, ts_qd)
% Position and rotation of actuator
% States
x   = s(1); % x-position of actuator
y   = s(2); % y-position of actuator
theta = s(3); % rotation of actuator

% Velocities
vx = s(4);
vy = s(5);
vr = s(6);

e = [x;y;theta] - ts_q; % error
e_d = [vx;vy;vr] - ts_qd;

D = 10*diag([1,1,1]);
K = 10*diag([5,5,5]);
% wr = -D*e_d-K*e - K_d*d_c;
wr = K_r*[ts_q; ts_qd]-[K_f K_a]*s - K_d*d_c;

== matlab function CDPR_simulation_w_motor/MATLAB Function3 ==
  data: states input; xdot output; v input; mp input; Izz input; E input; A input; ln_ik input; t output; lvec input; b input; wr output
function [xdot,t, wr] = dynamics(states,v,mp,Izz,E,A, ln_ik, lvec, b)
% States
x = states(1); % x-position of actuator
y = states(2); % y-position of actuator
theta = states(3); % rotation of actuator

vx = states(4);
vy = states(5);
vr = states(6);


% Length of unstretched cable rolled out.
ln_s = [states(7); states(8); states(9); states(10)];

% Compute tensions.
t = zeros(4,1);
for i=1:4
    t(i) = A*E*(ln_ik(i) - ln_s(i))/ln_s(i);
end

% Compute forces
F = zeros(2,4);
for i = 1:4
    F(:,i) = t(i)'*lvec(:,i)/ln_ik(i);
end

R = R_z(theta);
M = zeros(1,4);
for i = 1:4
    cross_prod = cross([R*b(:,i);0],[F(:,i);0]);
    M(i) = cross_prod(3);
end

F_res = F(:,1) + F(:,2) + F(:,3) + F(:,4);
M_res = M(1) + M(2) + M(3) + M(4);
wr = [F_res;M_res];

xdot = [vx;vy;vr;F_res(1)/mp;F_res(2)/mp-9.81;M_res/Izz;-v(1);-v(2);-v(3);-v(4)];

end

== matlab function CDPR_simulation_w_motor/Inverse kinematics/MATLAB Function4 ==
  data: q input; a input; ln output; b input
function ln = inverse_kinematics(q, a, b)
    x     = q(1);
    y     = q(2);
    theta = q(3);

    R = R_z(theta);
    
    ln = zeros(4,1);
    for i=1:4
        ln(i) = norm(a(:,i)-[x;y]-R*b(:,i),2);
    end
end

== matlab function CDPR_simulation_w_motor/Cable vector calculation/MATLAB Function5 ==
  data: q input; l_vec output; a input; b input
function l_vec = calculate_l_vec(q, a, b)
    r = q(1:2);
    theta = q(3);
    
    R = R_z(theta);

    l_vec = zeros(2,4);
    for i = 1:4
        l_vec(:,i) = a(:,i) - r - R*b(:,i);
    end
end

== matlab function CDPR_simulation_w_motor/Cable force model/Cable model ==
  data: fc output; t output; A input; E input; cable_states input; ln_ik input; lvec input
function [fc, t] = calculate_cable_forces(A, E, cable_states, ln_ik, lvec)
% Length of unstretched cable rolled out.
ln_s = [cable_states(1); 
        cable_states(2); 
        cable_states(3); 
        cable_states(4)];

% Calculate tensions
t = zeros(4,1);
for i=1:4
    t(i) = A*E*(ln_ik(i) - ln_s(i))/ln_s(i);
end

% Calculate forces
fc = zeros(2,4);
for i = 1:4
    fc(:,i) = t(i)'*lvec(:,i)/ln_ik(i);
end
